simulink model "trab1linearFTS"  (R2020a)
settings: Solver=VariableStepAuto  StartTime=0.0  StopTime=10.0  RelTol=1e-3
model workspace (MAT data in the model file):
  Caf = 1
  U = 1
  s = 1
settings Model: Creator=luang  LastModifiedBy=luang

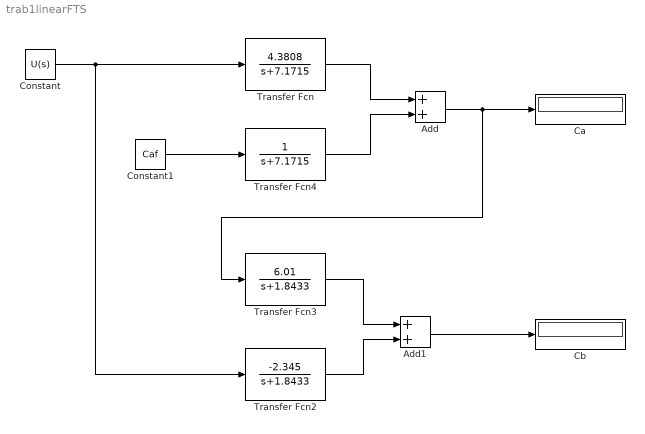
== system trab1linearFTS ==
  Add : Sum
  Add1 : Sum
  Ca : Display
  Cb : Display
  Constant : Constant  Value=U(s)
  Constant1 : Constant  Value=Caf
  Transfer Fcn : TransferFcn  Numerator=[4.3808]  Denominator=[1 7.1715]
  Transfer Fcn2 : TransferFcn  Numerator=[-2.345]  Denominator=[1 1.8433]
  Transfer Fcn3 : TransferFcn  Numerator=[6.01]  Denominator=[1 1.8433]
  Transfer Fcn4 : TransferFcn  Denominator=[1 7.1715]
  wires:
  Constant/1 -> Transfer Fcn2/1, Transfer Fcn/1
  Transfer Fcn2/1 -> Add1/2
  Transfer Fcn3/1 -> Add1/1
  Add/1 -> Transfer Fcn3/1, Ca/1
  Transfer Fcn/1 -> Add/1
  Transfer Fcn4/1 -> Add/2
  Constant1/1 -> Transfer Fcn4/1
  Add1/1 -> Cb/1
